simulink model "base_reference"  (R2019a)
settings: Solver=ode23tb  StartTime=0.0  StopTime=60  RelTol=1e-3
model workspace (MAT data in the model file):
  A_mu = 10
  AxlIxx = 62.3745166667
  AxlM = 160
  B_reff = 8.386
  BattCapInit = 26
  BattChargeMax = 32.5
  BattChrgMax = -80000
  BattDischrgMax = 80000
  BattTempBp = [243.1 253.1 263.1 273.1 283.1 298.1 313.1]
  BrkPrsMax = 5000000
  CapLUTBp = [0 0.01 0.02 0.03 0.04 0.05 0.06 0.07 0.08 0.09 0.1 0.11 ... (101 elements, 1x101)]
  CapSOCBp = [0 0.2 0.4 0.6 0.8 1]
  ChrgLmt_bpt = [1 1 1 1 1 1 1 1 0.7 0.35 0]
  Cps = 2
  Cz = 5565.2246438
  CzWhlAxl = 11490.971257
  DCT_Param : struct (value not decoded)
  DLCXref = [0 6 7 14 33.5 34 42 50 60]
  DLCYref = [0 0 -4.5 -4 -3.75 1.5 0.5 0 0]
  D_reff = 0.25826
  DischrgLmt_bpt = [0 0.35 0.7 1 1 1 1 1 1 1 1]
  Downshift_Speeds = [9.5625 12.9375 16.3125 19.6875 23.0625 26.4375 29.8125 33.1875 36.5625 39.9375 43.3125 46.6875 ... (28 elements, 4x7)]
  EV_current = 200
  EV_motion = [20 4 0.8]
  EV_sf = 2000
  Em = [2.8 3.228 3.284 3.361 3.408 3.427 3.472 3.477 3.493 3.504 3.516 3.528 ... (101 elements, 1x101)]
  EngRevLim = 7000
  F0z = [2886 2907]
  F0zWhlAxl = 2907
  Fs = 0
  Fv = 0.0025
  Hmax = 0.25
  Jcomp = 0.0227
  Ki = 251.3274
  Kisa = 346.6583
  Kp_d = 0.47149
  Kp_q = 0.52125
  Ksa = 85.4316
  Ksf = 1996.2651
  Kz = 52451.0065793
  KzWhlAxl = 138031.612078
  Ld = 0.0003752
  Ldq = [0.0003752 0.0004148]
  Lq = 0.0004148
  Mechanical = [0.0227 0.0025 0]
  MotMapEff = 0
  MotSpd = [0 1000 2000 2728.370453 3000 4000 5000 6000 7000 8000 9000 10000]
  MotTrq = [280 280 280 280 254.6479089 190.9859317 152.7887454 127.3239545 109.1348181 95.49296586 84.88263632 76.39437268]
  NCyl = 6
  Ndiff = 7.94
  Np = 2
  Ns = 96
  P = 4
  Pedal_Positions = [0.1 0.4 0.5 0.9]
  PolePairs = 4
  Pstd = 101325
  RInt = [0.008846 0.006389 0.004364 0.002031 0.001443 0.0005603 0.001028 0.009319 0.006554 0.004101 0.002563 0.001825 ... (42 elements, 7x6)]
  Rair = 287
  RegenBrkCutOff = [0 1]
  RegenBrkSpd_bpt = [5 9]
  Rm = 0.15
  Rs = 0.2
  SOC_bpt = [0 10 20 30 40 50 60 70 80 90 100]
  SUS : struct (value not decoded)
  T_eff_bp = [0 20 40 60 80 100 120 140 160 180 200 220 ... (15 elements, 1x15)]
  T_max = 120
  T_mtpa = [0 13.3131834767 26.6278836885 39.9456159322 53.2678926341 66.5962219318 79.9321062746 93.277041051 106.632513247 120.000000141]
  Tc = 0.02
  Trans : struct (value not decoded)
  Tstd = 293.15
  Upshift_Speeds = [12.9375 16.3125 19.6875 33 26.4375 29.8125 33.1875 52.5 39.9375 43.3125 46.6875 77.25 ... (28 elements, 4x7)]
  VEH : struct (value not decoded)
  V_o = 16.7
  V_xlow = 1
  Vd = 0.00346
  WH : struct (value not decoded)
  a = 1.4
  alpha_max = 1.5
  alpha_min = -1.5
  b = 1.8
  ba = 3.4029
  c_zo = 209651
  disk_abore = 0.05
  dt3D = 0.05
  efficiency_table = [85 85 85 85 85 85 85 85 85 85 85 85 ... (180 elements, 12x15)]
  epsilon = 0.1
  f_air = [0 0 0 0 0 0 0 0 0 0 0 0 ... (256 elements, 16x16)]
  f_co = [0 0 0 0 0 0 0 0 0 0 0 0 ... (256 elements, 16x16)]
  f_co2 = [0 0 0 0 0 0 0 0 0 0 0 0 ... (256 elements, 16x16)]
  f_eff = [352.135682859 352.135682859 320.724378192 303.655312657 295.930136708 291.240087194 291.240271258 291.240312459 291.240275452 291.240198499 291.240100781 291.240018769 ... (256 elements, 16x16)]
  f_fuel = [0 0 0 0 0 0 0 0 0 0 0 0 ... (256 elements, 16x16)]
  f_hc = [0 0 0 0 0 0 0 0 0 0 0 0 ... (256 elements, 16x16)]
  f_nox = [0 0 0 0 0 0 0 0 0 0 0 0 ... (256 elements, 16x16)]
  f_pm = [0 0 0 0 0 0 0 0 0 0 0 0 ... (256 elements, 16x16)]
  f_susp_axl_bp = [1 2]
  f_susp_dz_bp = [-0.325022776267 -0.315022776267 -0.305022776267 -0.205022776267 -0.105022776267 -0.00502277626717 0.0949772237328 0.194977223733 0.204977223733 0.214977223733]
  f_susp_dzdot_bp = [-3 -0.3 -0.2 -0.1 0 0.1 0.2 0.3 3]
  f_susp_fmz = [-144070.391448 -93629.24037 -75929.1118915 -20630.5828179 -15385.48216 -10140.3815021 -4895.28084414 349.819813785 -31916.3973792 18437.6709544 -83996.1993354 -33555.0482577 ... (43920 elements, 10x9x61x2x4)]
  f_susp_geom = [0 0 0 0 0 0 0 0 0 0 0 0 ... (3660 elements, 10x61x2x3)]
  f_susp_strgdelta_bp = [-0.523598775598 -0.506145483078 -0.488692190558 -0.471238898038 -0.453785605519 -0.436332312999 -0.418879020479 -0.401425727959 -0.383972435439 -0.366519142919 -0.349065850399 -0.331612557879 ... (61 elements, 1x61)]
  f_tbrake = [0 76.8593923996 105.140482948 131.533638111 157.926793274 176.658631717 176.65727296 176.656856686 176.656879077 176.657093756 176.657404516 176.65772406 ... (256 elements, 16x16)]
  f_tbrake_n_bpt = [0 649.519052838 912.419621844 1175.32019085 1438.22075986 1701.12132886 1964.02189787 2226.92246687 2489.82303588 2752.72360489 3015.62417389 3278.5247429 ... (16 elements, 1x16)]
  f_tbrake_t_bpt = [0 34.6410161514 61.0341713143 87.4273264773 113.82048164 140.213636803 166.606791966 192.999947129 219.393102292 245.786257455 272.179412618 298.572567781 ... (16 elements, 1x16)]
  f_texh = [766.752464599 766.752464599 786.17542386 801.679939032 884.591982581 910.574397722 910.571871054 910.570774534 910.570601632 910.570821151 910.571247242 910.571639815 ... (256 elements, 16x16)]
  f_twc_eff_co = [0.17 0.25 0.45 0.99 0.99 0.99 0.99]
  f_twc_eff_hc = [0.21 0.375 0.75 0.98 0.98 0.98 0.98]
  f_twc_eff_lam = [0.909090909 0.944055944 0.979020979 1 1.013986014 1.048951049 1.083916084]
  f_twc_eff_nox = [0.98 0.98 0.98 0.97 0.05 0.02 0]
  h = 0.134
  id_mtpa = [0 -0.114523352646 -0.457989076459 -1.03008464374 -1.83029075221 -2.85788367342 -4.11193850568 -5.59133329791 -7.29475400168 -9.22070020138]
  idq0 = [0 0]
  idq_limits = [-9.220699542 166.993501392 167.247872355]
  iq_mtpa = [0 18.5827440345 37.1633719111 55.7397734896 74.3098506185 92.871523015 111.422734008 129.961456105 148.485696337 166.993501356]
  lambda_pm = 0.1194
  mechanical = [0.0227 0.0025 0]
  mu_kinetic = 0.35
  numWheel = 4
  num_pads = 2
  omega_init = 0
  path : struct (value not decoded)
  pio = 220000
  power_max = 80000
  q_Fcx = 0
  q_Fz2 = 15.4
  q_Fzy = 0
  q_reo = 0.9974
  q_sx1 = -0.007764
  q_sx10 = 0.2824
  q_sx11 = 5.349
  q_sx12 = 0
  q_sx13 = 0
  q_sx14 = 0
  q_sx2 = 1.1915
  q_sx3 = 0.013948
  q_sx4 = 4.912
  q_sx5 = 1.02
  q_sx6 = 22.83
  q_sx7 = 0.7104
  q_sx8 = -0.023393
  q_sx9 = 0.6581
  q_sy1 = 0.00702
  q_sy2 = 0
  q_sy3 = 0.001515
  q_sy4 = 8.514e-05
  q_sy5 = 0
  q_sy6 = 0
  q_sy7 = 0.9008
  q_sy8 = -0.4089
  q_v1 = 0.0007742
  q_v2 = 0.04667
  r_Bx1 = 12.531
  r_Bx2 = 9.532
  r_Bx3 = 0
  r_By1 = 10.615
  r_By2 = 7.705
  r_By3 = 3.433e-06
  r_By4 = 0
  r_Cx1 = 1.019
  r_Cy1 = 1.0585
  r_Ex1 = -0.4487
  r_Ex2 = -0.4726
  r_Ey1 = 0.3132
  r_Ey2 = 7.63e-06
  r_Hx1 = 0.0002374
  r_Hy1 = 0.011646
  r_Hy2 = 7.63e-06
  r_Vy1 = 0.05654
  r_Vy2 = 7.63e-06
  r_Vy3 = 0
  r_Vy4 = 99.9
  r_Vy5 = 2
  r_Vy6 = 15.814
  r_o = 0.3135
  theta_init = 0
  torque_max = 280
  vehWidth = 2
  w = 1
  w_eff_bp = [0 1000 2000 2728.370453 3000 4000 5000 6000 7000 8000 9000 10000]
values from neighbouring files (symbols this model uses):
  VEH =     [PassVeh14DOF.mat]    (also in model2.mat; model_workspace_reference.mat)
undefined symbols (not defined in the file or in its folder): Disabled, Right
libraries: simulink x8, vehdynlibtire x8, vehdynlibsuspension x7, autolibutils x6, vehdynlibscenariocommon x5, sim3dlib x4, autolibmappedmotor x4, autolibshared x2, sharedtransform x2, vehdynlibviscommon x2, vehdynlibdriver x1, vehdynlibsteering x1
(part 2 of 8)

== system base_reference/Controllers ==
  Driver : Inport
  Vehicle_loop : Inport  Port=2
  Accel Pedal to Traction Wheel Torque Request : Subsystem
  Active Differential Control : Subsystem  VariantControlMode=Label  Variant=on  LabelModeActiveChoice=0
  Battery Management System : Subsystem
  Brake Pedal to Total Braking Pressure Request : Subsystem
  Bus Creator2 : BusCreator  Inputs=1
  Bus Creator3 : BusCreator  Inputs=3
  Bus Creator4 : BusCreator  Inputs=1
  Bus Selector : BusSelector  OutputSignals=ElecFdbk.BattSoc,Driveline.EngSpd,Body.r
  Bus Selector3 : BusSelector  OutputSignals=Steer,Accel,Brake
  Constant : Constant  Value=0
  Max : MinMax  Function=max  Inputs=2
  Motor Torque Arbitration and Power Management : Subsystem
  Regen Braking Control : Subsystem  VariantControlMode=Label  Variant=on  VariantControl=(default)  LabelModeActiveChoice=Variant
  Controller : Outport
  wires:
  Driver/1 -> Bus Selector3/1
  Max/1 -> Bus Creator3/1  "acc"
  Bus Creator2/1 -> Bus Creator3/2  "Brake"
  Bus Creator3/1 -> Controller/1  "Controller"
  Active Differential Control/1(DiffPrsCmd) -> Bus Creator4/1  "PrsCmd"
  Bus Selector3/1 -> Active Differential Control/2(Steer)  "<Steer>"
  Active Differential Control/2(TrqCmd) -> [DiffTrqCmd]
  Battery Management System/1(BattPwrDischrgLmt) -> Motor Torque Arbitration and Power Management/3(BattPwrDisChrgLmt)  "BattPwrDischrgLmt"
  Regen Braking Control/1(" MotTrqCmdRegen") -> Motor Torque Arbitration and Power Management/6(MotTrqCmdRegen)  "MotTrqCmdRegen"
  [MotSpd] -> Motor Torque Arbitration and Power Management/5(MotSpd)
  Bus Selector/2 -> Regen Braking Control/3("MotSpd "), [MotSpd], Regen Braking Control/2("VehSpd ")  "<EngSpd>"
  Accel Pedal to Traction Wheel Torque Request/1(TrqCmd) -> Motor Torque Arbitration and Power Management/1(MotTrqCmdTrac)
  Battery Management System/2(BattPwrChrgLmt) -> Motor Torque Arbitration and Power Management/4("BattPwrChrgLmt ")  "BattPwrChrgLmt"
  Bus Selector3/3 -> Brake Pedal to Total Braking Pressure Request/1(DecelPdl)  "<Brake>"
  Regen Braking Control/2(" BrkCmd") -> Bus Creator2/1  "BrkCmd"
  Constant/1 -> Brake Pedal to Total Braking Pressure Request/2(Park)
  [MotSpd] -> Accel Pedal to Traction Wheel Torque Request/2(MotSpd)
  Bus Selector/1 -> Battery Management System/1(SOC), Regen Braking Control/1("BattSoc ")  "<BattSoc>"
  Brake Pedal to Total Braking Pressure Request/1(BrkPrsReq) -> Regen Braking Control/4("BrkPrsReq ")
  [AccelPdl] -> Motor Torque Arbitration and Power Management/2(AccelPdl)
  Bus Selector3/2 -> [AccelPdl], Accel Pedal to Traction Wheel Torque Request/1(AccelPdl)  "<Accel>"
  Bus Creator4/1 -> Bus Creator3/3  "Diff"
  Vehicle_loop/1 -> Bus Selector/1
  Bus Selector/3 -> Active Differential Control/1(YawRate)  "<r>"
  [DiffTrqCmd] -> Max/1
  Motor Torque Arbitration and Power Management/1(MotTrqCmdFinal) -> Max/2  "MotTrqCmd4"

== system base_reference/Driver Commands ==
  VehRef : Inport
  VehFdbk : Inport  Port=2
  AccelGround : Ground
  BrakeGround : Ground
  Driver Commands : Subsystem  VariantControlMode=Label  Variant=on  VariantControl=Variant1  LabelModeActiveChoice=1  AllowZeroVariantControls=on
  GearGround : Ground
  SteerGround : Ground
  Driver : Outport
  wires:
  VehRef/1 -> Driver Commands/1(VehRef)
  VehFdbk/1 -> Driver Commands/2(VehFdbk)
  Driver Commands/1(" Driver") -> Driver/1
  SteerGround/1 -> Driver Commands/3(SteerCmd)
  AccelGround/1 -> Driver Commands/4(Accel)
  BrakeGround/1 -> Driver Commands/5(Brake)
  GearGround/1 -> Driver Commands/6(Gear)

== system base_reference/Environment ==
  Bus Creator1 : BusCreator  Inputs=4
  Constant3 : Constant  Value=0
  Constant4 : Constant  Value=0
  Constant5 : Constant  Value=0
  Constant6 : Constant  Value=300
  Constant7 : Constant  Value=101325
  Friction : Constant  Value=ones(4,1).*1
  Ground Feedback : Subsystem  VariantControlMode=Label  Variant=on  LabelModeActiveChoice=0
  Vector Concatenate : Concatenate  NumInputs=3
  Env : Outport
  wires:
  Constant5/1 -> Vector Concatenate/3  "Z"
  Vector Concatenate/1 -> Bus Creator1/3  "Wind"
  Constant3/1 -> Vector Concatenate/1  "X"
  Constant4/1 -> Vector Concatenate/2  "Y"
  Ground Feedback/1(Ground) -> Bus Creator1/4  "Gnd"
  Bus Creator1/1 -> Env/1
  Friction/1 -> Ground Feedback/1(Friction)
  Constant6/1 -> Bus Creator1/1  "Temp"
  Constant7/1 -> Bus Creator1/2  "Baro"

== system base_reference/Passenger Vehicle ==
  Env : Inport
  Operator : Inport  Port=2
  Cntrl : Inport  Port=3
  Bus Creator2 : BusCreator  Inputs=4
  Subsystem : Subsystem
  Subsystem1 : Subsystem
  Subsystem2 : Subsystem
  Subsystem4 : Subsystem
  Subsystem5 : Subsystem
  Subsystem6 : Subsystem
  VehFdbk : Outport
  wires:
  Bus Creator2/1 -> VehFdbk/1
  Env/1 -> Subsystem2/4(Env), Subsystem/1(Env)
  Subsystem1/1(Driveline) -> [Driveline], Bus Creator2/1  "Driveline"
  Subsystem5/1(WhlAng) -> Subsystem1/1(WhlAng)
  Operator/1 -> Subsystem2/2(SteerCmd)
  Cntrl/1 -> Subsystem2/1(Cntrl)
  Subsystem2/1(Steer) -> Subsystem5/1(SteerHWCmd)
  Subsystem2/2(brake) -> Subsystem5/2(BrkPrsCmd)
  Subsystem4/2(Wheels) -> Bus Creator2/4, [Wheels]  "Wheels"
  [Driveline] -> Subsystem/2(Driveline)
  [Wheels] -> Subsystem2/3(Wheels)
  Subsystem6/15(dzWheel) -> Subsystem4/15(dzWheel)
  Subsystem6/3(CgXYZdot) -> Subsystem4/3(CgXYZdot)
  Subsystem6/1(Cgxyzdot) -> Subsystem4/1(Cgxyzdot)
  Subsystem6/5(pqr) -> Subsystem4/5(pqr)
  Subsystem6/14(YWheel) -> Subsystem4/14(YWheel)
  Subsystem6/7(Beta) -> Subsystem4/7(Beta)
  Subsystem6/6(Cgaxyz) -> Subsystem4/6(Cgaxyz)
  Subsystem6/8(GeomXYZ) -> Subsystem4/8(GeomXYZ)
  Subsystem6/4(angles) -> Subsystem4/4(angles)
  Subsystem6/11(kappa) -> Subsystem4/11(kappa)
  Subsystem6/13(XWheel) -> Subsystem4/13(XWheel)
  Subsystem6/2(CgXYZ) -> Subsystem4/2(CgXYZ)
  Subsystem6/9(GeomXYZdot) -> Subsystem4/9(GeomXYZdot)
  Subsystem6/10(omega) -> Subsystem4/10(omega)
  Subsystem6/12(alpha) -> Subsystem4/12(alpha)
  Subsystem5/2(BrkPrs) -> Subsystem1/2(BrkPrs)
  Subsystem5/5(BattSoc) -> Subsystem1/5(BattSoc)
  Subsystem5/6(BattPwr) -> Subsystem1/6(BattPwr)
  Subsystem5/7(BattCrnt) -> Subsystem1/7(BattCrnt)
  Subsystem2/4(acc) -> Subsystem5/4("acc ")
  Subsystem5/3(AxlTrq) -> Subsystem1/3(AxlTrq)
  Subsystem5/4(Motor_speed) -> Subsystem1/4(EngSpd)
  Subsystem2/5(amb_temp) -> Subsystem5/5(AmbTmp)
  Subsystem2/3(omega) -> Subsystem5/3(speed_wheel)
  Subsystem1/2(ElecFdbk) -> Bus Creator2/2  "ElecFdbk"
  Subsystem4/1(Chassis) -> Bus Creator2/3  "Body"
  Subsystem/1(Wind) -> Subsystem6/1(WindXYZ)
  Subsystem/2(Gnd) -> Subsystem6/2(Ground)
  Subsystem/3(mu) -> Subsystem6/3(Friction)
  Subsystem/4(WhlAng) -> Subsystem6/4(WheelAngle)
  Subsystem/5(AxleTrq) -> Subsystem6/5(AxleTrq)
  Subsystem/6(BrkPrs) -> Subsystem6/6(BrkPrs)

== system base_reference/Reference Generator ==
  "VehFdbk " : Inport
  3D Engine : Subsystem  VariantControlMode=Label  Variant=on  LabelModeActiveChoice=0  mask(3D Engine){engine3D=Disabled, SceneDesc=Open surface, dt3D=dt3D, defaultPos=User-specified, X_o=X_o, Y_o=Y_o, Z_o=Z_o, phi_o=phi_o, theta_o=theta_o, psi_o=psi_o}
      mask prompts: engine3D "3D Engine"; SceneDesc "Scene:"; dt3D "Engine frame rate, dt3D [s]:"; X_o "Initial longitudinal position, X_o [m]:"; Y_o "Initial lateral position, Y_o [m]:"; Z_o "Initial vertical position, Z_o [m]:"; phi_o "Initial roll angle, phi_o [rad]:"; theta_o "Initial pitch angle, theta_o [rad]:"; psi_o "Initial yaw angle, psi_o [rad]:"
      mask help: This subsystem contains the interface blocks which permit the display of the vehicle in the 3D virtual environment. Enable it to view the simulation progress, disable it to inhibit the display.
      mask init:
      | switch get_param(gcb,'engine3D')
      |     case 'Disabled'
      |         set_param(gcb,'OverrideUsingVariant','0')
      |         try
      |             set_param([bdroot '/Environment/Ground Feedback'],'OverrideUsingVariant','0')
      |         catch
      |             disp('Warning: No ground feedback sensor not set')
      |         end
      |     case 'Enabled'
      |         set_param(gcb,'OverrideUsingVariant','1')
      |         try
      |             set_param([bdroot '/Environment/Ground Feedback'],'OverrideUsingVariant','1')
      |         catch
      |             disp('Warning: No ground feedback sensor not set')
      |         end
      |     otherwise
      |         set_param(gcb,'OverrideUsingVariant','0')
      | end
      settings: AttributesFormatString=|
      | %<SceneDesc>
      | %<engine3D>
      mask Help: eval('vdynblkshelp(''vdynblks3dengine'')');
      mask TypeOptions engine3D: Enabled | Disabled
      mask Callback engine3D:
      | switch get_param(gcb,'engine3D')
      |     case 'Disabled'
      |         set_param(gcb,'OverrideUsingVariant','0')
      |     case 'Enabled'
      |        set_param(gcb,'OverrideUsingVariant','1')
      |     otherwise
      |        set_param(gcb,'OverrideUsingVariant','0')
      | end
      mask TypeOptions SceneDesc:
      | 3D Engine/Simulation 3D Engine
      | 1/SceneDesc
      mask Callback SceneDesc: [~] = vdynblks3Dsceneconfig(gcb);
      mask TypeOptions defaultPos: Recommended for scene | User-specified
      mask DialogControl engineConfig Prompt: 3D Engine Settings
      mask DialogControl posSetup Prompt: Initial vehicle position
      mask DialogControl posSetupDesc Prompt: To use these initial vehicle positions, first Apply the initial values and then click Update the model workspaces with the initial values.
      mask DialogControl setModelPos Prompt: Update model workspaces with initial values
      mask DialogControl setModelPos Callback: [~] = vdynblksmdlWSconfig(gcb);
      mask Display: disp('3D Engine')
  Reference Generator : Subsystem  VariantControlMode=Label  Variant=on  VariantControl=Variant1  LabelModeActiveChoice=4
  " Vis" : Outport
  " Ref" : Outport  Port=2
  " Fdbk" : Outport  Port=3
  wires:
  "VehFdbk "/1 -> 3D Engine/1(VehFdbk), Reference Generator/1("VehFdbk ")
  Reference Generator/1(" Vis") -> " Vis"/1
  Reference Generator/2(" Ref") -> " Ref"/1
  Reference Generator/3(" Fdbk") -> " Fdbk"/1

== system base_reference/Visualization ==
  note: Vehicle Response
  note: Driver Commands
  Vis : Inport
  Cntrl : Inport  Port=2
  VehFdbk : Inport  Port=3
  Acceleration Cmd : LinearGaugeBlock  LabelPosition=Hide  ScaleMax=1  TickInterval=0.20000000000000001
  Brake Cmd : LinearGaugeBlock  LabelPosition=Hide  ScaleMax=1  TickInterval=0.20000000000000001
  Bus Selector : BusSelector  OutputSignals=Body.xdot,Body.ay
  Bus Selector2 : BusSelector  OutputSignals=Accel,Brake,Steer
  Engine Tach [rpm] : CircularGaugeBlock  LabelPosition=Hide  ScaleMax=8000  TickInterval=1000
  Handwheel Angle [deg] : SemiCircularGaugeBlock  LabelPosition=Hide  ScaleMin=-300  ScaleMax=300  TickInterval=60
  ISO 15037-1:2006 : Subsystem  StopFcn=|  VariantControlMode=Label  Variant=on  LabelModeActiveChoice=0  mask(ISO 15037-1:2006){Measurement=Disabled}
      | switch get_param(gcb,'Measurement')
      |     case 'Enabled'
      |        p=slproject.getCurrentProject;
      |        projectRoot=p.RootFolder;
      |        SySFolder=fullfile(projectRoot, 'System');
      |        Simulink.sdi.loadView([SySFolder filesep 'ISO15037_1_2006E.mldatx']);
      |        Simulink.sdi.view;
      | end
      mask prompts: Measurement "ISO Measurements"
      mask help: Enables display of ISO 15037-1:2006 standard measurement signals in the Simulation Data Inspector.
      mask init:
      | switch get_param(gcb,'Measurement')
      |     case 'Disabled'
      |         set_param(gcb,'OverrideUsingVariant','0')
      |     case 'Enabled'
      |        set_param(gcb,'OverrideUsingVariant','1')
      |     otherwise
      |        set_param(gcb,'OverrideUsingVariant','0')
      | end
      settings: AttributesFormatString=%<Measurement>
      mask Help: eval('vdynblkshelp(''iso15037'')');
      mask TypeOptions Measurement: Enabled | Disabled
      mask Callback Measurement:
      | switch get_param(gcb,'Measurement')
      |     case 'Disabled'
      |         set_param(gcb,'OverrideUsingVariant','0')
      |     case 'Enabled'
      |        set_param(gcb,'OverrideUsingVariant','1')
      |     otherwise
      |        set_param(gcb,'OverrideUsingVariant','0')
      | end
      mask Display: disp('ISO 15037-1:2006')
  Lateral Acceleration [g] : SemiCircularGaugeBlock  LabelPosition=Hide  ScaleMin=-1  ScaleMax=1  TickInterval=0.5
  Rate Transition1 : RateTransition  Deterministic=off  OutPortSampleTime=.1
  Rate Transition2 : RateTransition  Deterministic=off  OutPortSampleTime=.1
  Scope Type : Subsystem  VariantControlMode=Label  Variant=on  VariantControl=Variant1  LabelModeActiveChoice=2
  Signal Specification : SignalSpecification  Unit=deg
  Signal Specification1 : SignalSpecification  Unit=mph
  Speed [mph] : CircularGaugeBlock  LabelPosition=Hide  TickInterval=10
  Steer vs Ay : simulink/Sinks/XY Graph  Commented=on  xmin=-300  xmax=300  ymin=-1.5  ymax=1.5  st=.1
  "Steer, Velocity, Lat Accel" : Scope  NumInputPorts=3
  Terminator : Terminator
  Terminator1 : Terminator
  Terminator2 : Terminator
  Unit Conversion1 : UnitConversion
  Unit Conversion2 : UnitConversion
  Vehicle XY Plotter : Subsystem  VariantControlMode=Label  Variant=on  VariantControl=Variant1  LabelModeActiveChoice=1
  wires:
  Signal Specification/1 -> Rate Transition1/1, "Steer, Velocity, Lat Accel"/1  "SteerAngle"
  Bus Selector/2 -> Rate Transition2/1, "Steer, Velocity, Lat Accel"/3  "<ay>"
  Bus Selector/1 -> "Steer, Velocity, Lat Accel"/2, Unit Conversion1/1  "<xdot>"
  Unit Conversion2/1 -> Signal Specification/1
  Unit Conversion1/1 -> Signal Specification1/1
  Signal Specification1/1 -> Terminator/1  "xdot_mph"
  Bus Selector2/3 -> Unit Conversion2/1  "<Steer>"
  Rate Transition1/1 -> Steer vs Ay/1
  Rate Transition2/1 -> Steer vs Ay/2
  Bus Selector2/1 -> Terminator1/1  "<Accel>"
  Bus Selector2/2 -> Terminator2/1  "<Brake>"
  VehFdbk/1 -> ISO 15037-1:2006/1(VehFdbk), Scope Type/1("VehFdbk "), Vehicle XY Plotter/1("VehFdbk "), Bus Selector/1  "VehFdbk"
  Cntrl/1 -> ISO 15037-1:2006/2(Cntrl), Scope Type/2(Cntrl), Bus Selector2/1
  Vis/1 -> Scope Type/3("Vis ")
  Scope Type/1(" Ref") -> Vehicle XY Plotter/2("Ref ")

== system base_reference/Controllers/Accel Pedal to Traction Wheel Torque Request ==
  note: Convert Accelerator Pedal Position to Torque Command
      | using Motor Torque Speed Curve
  AccelPdl : Inport
  MotSpd : Inport  Port=2
  MaxMotTrqVsSpd : Lookup_n-D  NumberOfTableDimensions=1  BreakpointsForDimension1=MotSpd  Table=MotTrq  ExtrapMethod=Clip  UseLastTableValue=on  InternalRulePriority=Speed  OutDataTypeStr=Inherit: Inherit from 'Table data'  RndMeth=Simplest  InputSameDT=on
  Product1 : Product
  rads_to_rpm : Gain  Gain=30/pi
  TrqCmd : Outport
  wires:
  Product1/1 -> TrqCmd/1
  MaxMotTrqVsSpd/1 -> Product1/2
  AccelPdl/1 -> Product1/1
  MotSpd/1 -> rads_to_rpm/1
  rads_to_rpm/1 -> MaxMotTrqVsSpd/1

== system base_reference/Controllers/Active Differential Control ==
  note: 1) Add Subsystem or Model blocks as valid variant choices.
      | 2) You cannot connect blocks at this level. At simulation, connectivity is automatically
      | determined, based on the active variant and port name matching.
  YawRate : Inport
  Steer : Inport  Port=2
  No Control : Subsystem  VariantControl=0
  Rear Diff Controller : Subsystem  VariantControl=1
  DiffPrsCmd : Outport
  TrqCmd : Outport  Port=2

== system base_reference/Controllers/Battery Management System ==
  note: Behaviorial BMS System. Limits battery charge / discharge power based on SOC.
      |
      | Charge/Discharge Limits and curves can be adjusted if using a larger battery pack
      | or motor power is changed.
  SOC : Inport
  ChrgLmt : Lookup_n-D  NumberOfTableDimensions=1  BreakpointsForDimension1=SOC_bpt  Table=ChrgLmt_bpt  ExtrapMethod=Clip  UseLastTableValue=on  InternalRulePriority=Speed  RndMeth=Simplest  InputSameDT=on
  DischrgLmt : Lookup_n-D  NumberOfTableDimensions=1  BreakpointsForDimension1=SOC_bpt  Table=DischrgLmt_bpt  ExtrapMethod=Clip  UseLastTableValue=on  InternalRulePriority=Speed  RndMeth=Simplest  InputSameDT=on
  MaxChrg : Constant  Value=BattChrgMax
  MaxDischrg : Constant  Value=BattDischrgMax
  Product : Product
  Product1 : Product
  BattPwrDischrgLmt : Outport
  BattPwrChrgLmt : Outport  Port=2
  wires:
  SOC/1 -> DischrgLmt/1, ChrgLmt/1
  MaxChrg/1 -> Product1/2
  MaxDischrg/1 -> Product/2
  Product/1 -> BattPwrDischrgLmt/1
  Product1/1 -> BattPwrChrgLmt/1
  ChrgLmt/1 -> Product1/1
  DischrgLmt/1 -> Product/1

== system base_reference/Controllers/Brake Pedal to Total Braking Pressure Request ==
  note: Converts Brake Pedal Position to Brake Pressure Request
  DecelPdl : Inport
  Park : Inport  Port=2
  Constant : Constant  Value=BrkPrsMax
  Constant1 : Constant
  Product1 : Product
  Switch : Switch  Criteria=u2 > Threshold
  BrkPrsReq : Outport
  wires:
  Constant/1 -> Product1/2
  Switch/1 -> Product1/1
  DecelPdl/1 -> Switch/3
  Constant1/1 -> Switch/1
  Product1/1 -> BrkPrsReq/1
  Park/1 -> Switch/2

== system base_reference/Controllers/Motor Torque Arbitration and Power Management ==
  MotTrqCmdTrac : Inport
  AccelPdl : Inport  Port=2
  BattPwrDisChrgLmt : Inport  Port=3
  "BattPwrChrgLmt " : Inport  Port=4
  MotSpd : Inport  Port=5
  MotTrqCmdRegen : Inport  Port=6
  Accel Decel Switch : Switch  Criteria=u2 > Threshold
  Compare To Constant : simulink/Logic and Bit Operations/Compare To Constant  relop=>  const=0  OutDataTypeStr=boolean
  Power Management : Subsystem
  MotTrqCmdFinal : Outport
  wires:
  AccelPdl/1 -> Compare To Constant/1
  MotTrqCmdRegen/1 -> Accel Decel Switch/3
  MotTrqCmdTrac/1 -> Accel Decel Switch/1
  Power Management/1(MotTrqCmdFinal) -> MotTrqCmdFinal/1
  Accel Decel Switch/1 -> Power Management/4(MotTrqCmd)
  BattPwrDisChrgLmt/1 -> Power Management/1(BattPwrDischrgLmt)
  "BattPwrChrgLmt "/1 -> Power Management/2(BattPwrChrgLmt)
  MotSpd/1 -> Power Management/3(MotSpd)
  Compare To Constant/1 -> Accel Decel Switch/2

== system base_reference/Controllers/Regen Braking Control ==
  "BattSoc " : Inport
  "VehSpd " : Inport  Port=2
  "MotSpd " : Inport  Port=3
  "BrkPrsReq " : Inport  Port=4
  Parallel Regen Braking : Subsystem  InitFcn=%[~]=autosharedicon('autolibutils',gcb,0);  VariantControl=(default)
  Series Regen Braking : Subsystem  InitFcn=%[~]=autosharedicon('autolibutils',gcb,0);  VariantControl=Variant
  " MotTrqCmdRegen" : Outport
  " BrkCmd" : Outport  Port=2

== system base_reference/Driver Commands/Driver Commands ==
  VehRef : Inport
  VehFdbk : Inport  Port=2
  SteerCmd : Inport  Port=3
  Accel : Inport  Port=4
  Brake : Inport  Port=5
  Gear : Inport  Port=6
  Longitudinal Driver : Subsystem  VariantControl=0
  Open Loop Constant Radius : Subsystem  VariantControl=2
  Predictive Driver : Subsystem  VariantControl=1
  " Driver" : Outport

== system base_reference/Environment/Ground Feedback ==
  note: 1) Add Subsystem or Model blocks as valid variant choices.
      | 2) You cannot connect blocks at this level. At simulation, connectivity is automatically
      | determined, based on the active variant and port name matching.
  Friction : Inport
  3D Engine : Subsystem  VariantControl=1
  Constant : Subsystem  VariantControl=0
  Ground : Outport

== system base_reference/Passenger Vehicle/Subsystem ==
  Env : Inport
  Driveline : Inport  Port=2
  Bus Selector1 : BusSelector  OutputSignals=Gnd.z.G_FL_z,Gnd.z.G_FR_z,Gnd.z.G_RL_z,Gnd.z.G_RR_z
  Bus Selector2 : BusSelector  OutputSignals=Wind
  Bus Selector3 : BusSelector  OutputSignals=Gnd.mu.mu_FL,Gnd.mu.mu_FR,Gnd.mu.mu_RL,Gnd.mu.mu_RR
  Bus Selector4 : BusSelector  OutputSignals=WhlAng,AxlTrq,BrkPrs
  Vector Concatenate : Concatenate  NumInputs=4
  Vector Concatenate1 : Concatenate  NumInputs=4
  Wind : Outport
  Gnd : Outport  Port=2
  mu : Outport  Port=3
  WhlAng : Outport  Port=4
  AxleTrq : Outport  Port=5
  BrkPrs : Outport  Port=6
  wires:
  Env/1 -> Bus Selector3/1, Bus Selector1/1, Bus Selector2/1
  Bus Selector2/1 -> Wind/1  "<Wind>"
  Bus Selector3/1 -> Vector Concatenate/1  "<mu_FL>"
  Bus Selector3/2 -> Vector Concatenate/2  "<mu_FR>"
  Bus Selector3/3 -> Vector Concatenate/3  "<mu_RL>"
  Bus Selector3/4 -> Vector Concatenate/4  "<mu_RR>"
  Vector Concatenate/1 -> mu/1
  Bus Selector1/1 -> Vector Concatenate1/1  "<G_FL_z>"
  Bus Selector1/2 -> Vector Concatenate1/2  "<G_FR_z>"
  Bus Selector1/3 -> Vector Concatenate1/3  "<G_RL_z>"
  Bus Selector1/4 -> Vector Concatenate1/4  "<G_RR_z>"
  Vector Concatenate1/1 -> Gnd/1
  Driveline/1 -> Bus Selector4/1
  Bus Selector4/2 -> AxleTrq/1  "<AxlTrq>"
  Bus Selector4/1 -> WhlAng/1  "<WhlAng>"
  Bus Selector4/3 -> BrkPrs/1  "<BrkPrs>"

== system base_reference/Passenger Vehicle/Subsystem1 ==
  WhlAng : Inport
  BrkPrs : Inport  Port=2
  AxlTrq : Inport  Port=3
  EngSpd : Inport  Port=4
  BattSoc : Inport  Port=5
  BattPwr : Inport  Port=6
  BattCrnt : Inport  Port=7
  Bus Creator1 : BusCreator  Inputs=4
  Bus Creator3 : BusCreator  Inputs=4
  Driveline : Outport
  ElecFdbk : Outport  Port=2
  wires:
  Bus Creator1/1 -> Driveline/1  "Driveline"
  AxlTrq/1 -> Bus Creator1/2, Bus Creator3/4  "AxlTrq"
  WhlAng/1 -> Bus Creator1/1  "WhlAng"
  EngSpd/1 -> Bus Creator1/4  "EngSpd"
  BrkPrs/1 -> Bus Creator1/3  "BrkPrs"
  BattCrnt/1 -> Bus Creator3/3
  BattPwr/1 -> Bus Creator3/2
  BattSoc/1 -> Bus Creator3/1
  Bus Creator3/1 -> ElecFdbk/1  "ElecFdbk"

== system base_reference/Passenger Vehicle/Subsystem2 ==
  Cntrl : Inport
  SteerCmd : Inport  Port=2
  Wheels : Inport  Port=3
  Env : Inport  Port=4
  Bus Selector1 : BusSelector  OutputSignals=Steer
  Bus Selector2 : BusSelector  OutputSignals=omega
  Bus Selector3 : BusSelector  OutputSignals=Brake,acc
  Bus Selector4 : BusSelector  OutputSignals=Temp
  Steer : Outport
  brake : Outport  Port=2
  omega : Outport  Port=3
  acc : Outport  Port=4
  amb_temp : Outport  Port=5
  wires:
  Cntrl/1 -> Bus Selector3/1
  SteerCmd/1 -> Bus Selector1/1
  Wheels/1 -> Bus Selector2/1
  Bus Selector2/1 -> omega/1  "<omega>"
  Bus Selector3/1 -> brake/1  "<Brake>"
  Bus Selector1/1 -> Steer/1  "<Steer>"
  Bus Selector3/2 -> acc/1  "<acc>"
  Bus Selector4/1 -> amb_temp/1  "<Temp>"
  Env/1 -> Bus Selector4/1

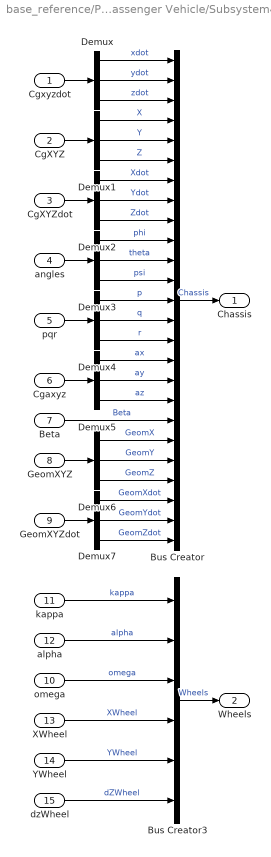
== system base_reference/Passenger Vehicle/Subsystem4 ==
  Cgxyzdot : Inport
  CgXYZ : Inport  Port=2
  CgXYZdot : Inport  Port=3
  angles : Inport  Port=4
  pqr : Inport  Port=5
  Cgaxyz : Inport  Port=6
  Beta : Inport  Port=7
  GeomXYZ : Inport  Port=8
  GeomXYZdot : Inport  Port=9
  omega : Inport  Port=10
  kappa : Inport  Port=11
  alpha : Inport  Port=12
  XWheel : Inport  Port=13
  YWheel : Inport  Port=14
  dzWheel : Inport  Port=15
  Bus Creator : BusCreator  Inputs=25
  Bus Creator3 : BusCreator  Inputs=6
  Demux{,1..7} (8 alike) : Demux  Outputs=3
  Chassis : Outport
  Wheels : Outport  Port=2
  wires:
  Bus Creator/1 -> Chassis/1  "Chassis"
  omega/1 -> Bus Creator3/3  "omega"
  dzWheel/1 -> Bus Creator3/6  "dZWheel"
  kappa/1 -> Bus Creator3/1  "kappa"
  Bus Creator3/1 -> Wheels/1  "Wheels"
  YWheel/1 -> Bus Creator3/5  "YWheel"
  XWheel/1 -> Bus Creator3/4  "XWheel"
  alpha/1 -> Bus Creator3/2  "alpha"
  Cgxyzdot/1 -> Demux/1
  CgXYZ/1 -> Demux1/1
  CgXYZdot/1 -> Demux2/1
  angles/1 -> Demux3/1
  pqr/1 -> Demux4/1
  Cgaxyz/1 -> Demux5/1
  GeomXYZdot/1 -> Demux7/1
  GeomXYZ/1 -> Demux6/1
  Demux/1 -> Bus Creator/1  "xdot"
  Demux/2 -> Bus Creator/2  "ydot"
  Demux/3 -> Bus Creator/3  "zdot"
  Demux1/1 -> Bus Creator/4  "X"
  Demux1/2 -> Bus Creator/5  "Y"
  Demux1/3 -> Bus Creator/6  "Z"
  Demux2/1 -> Bus Creator/7  "Xdot"
  Demux2/2 -> Bus Creator/8  "Ydot"
  Demux2/3 -> Bus Creator/9  "Zdot"
  Demux3/1 -> Bus Creator/10  "phi"
  Demux3/2 -> Bus Creator/11  "theta"
  Demux3/3 -> Bus Creator/12  "psi"
  Demux4/1 -> Bus Creator/13  "p"
  Demux4/2 -> Bus Creator/14  "q"
  Demux4/3 -> Bus Creator/15  "r"
  Demux5/1 -> Bus Creator/16  "ax"
  Demux5/2 -> Bus Creator/17  "ay"
  Demux5/3 -> Bus Creator/18  "az"
  Beta/1 -> Bus Creator/19  "Beta"
  Demux6/1 -> Bus Creator/20  "GeomX"
  Demux6/2 -> Bus Creator/21  "GeomY"
  Demux6/3 -> Bus Creator/22  "GeomZ"
  Demux7/1 -> Bus Creator/23  "GeomXdot"
  Demux7/2 -> Bus Creator/24  "GeomYdot"
  Demux7/3 -> Bus Creator/25  "GeomZdot"

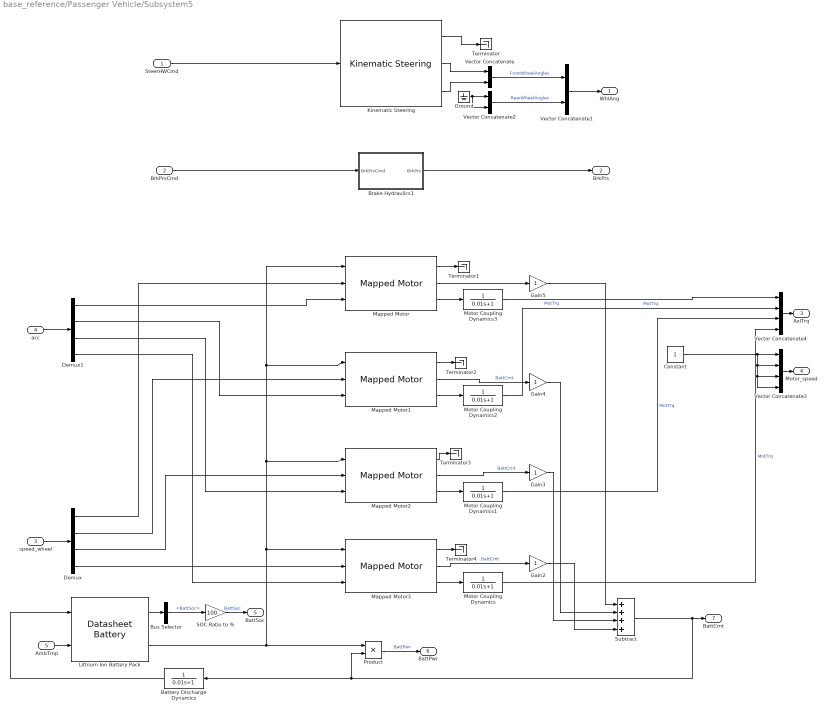
== system base_reference/Passenger Vehicle/Subsystem5 ==
  SteerHWCmd : Inport
  BrkPrsCmd : Inport  Port=2  PortDimensions=4
  speed_wheel : Inport  Port=3
  "acc " : Inport  Port=4
  AmbTmp : Inport  Port=5
  Battery Discharge Dynamics : TransferFcn  Denominator=[0.01 1]
  Brake Hydraulics1 : Subsystem
  Bus Selector : BusSelector  OutputSignals=BattSoc
  Constant : Constant
  Demux : Demux
  Demux1 : Demux
  Gain{2..5} (4 alike) : Gain
  Ground : Ground
  Kinematic Steering : vehdynlibsteering/Kinematic Steering  StrgType=Ackerman  StrgRatioType=Constant  Loc=Front  NrmlFctr=1  TrckWdth=1.922  WhlBase=(1.515+1.504)  Db=0  StrgRng=3*pi  StrgAngBpts="[-6.2832   -5.0265   -3.7699   -2.5133   -1.2566         0    1.2566    2.5133    3.7699    5.0265    6.2832]"  StrgRatioTbl=|  StrgRatio=18  StrgArmLngth=0.1  RckCsLngth=0.5  TieRodLngth=0.248128028933392  D=0.2  PnnRadius=0.0057  PnnRadiusTbl="[0.0055    0.0055    0.0056    0.0057    0.0057    0.0057    0.0057    0.0057    0.0056    0.0055    0.0055]"  RodLngth=0.1  ParaArmLngth=0.9  aMode=2
      | [13.5000   13.3750   13.2500   13.1250   13.0000   13.0000   13.0000   13.1250   13.2500   13.3750   13.5000
      | ]
      settings: SourceProductName=Vehicle Dynamics Blockset
  Lithium Ion Battery Pack : autolibdatasheetbattery/Datasheet Battery  CapacityCtrl=Parameter  OutputVlt=Unfiltered  BattChargeMax=BattChargeMax  Em=Em  CapLUTBp=CapLUTBp  RInt=RInt  BattTempBp=BattTempBp  CapSOCBp=CapSOCBp  Ns=Ns  Np=Np  BattCapInit=BattCapInit  Tc=1/1000  Vinit=3.75*72  RefBlkName='autolibdatasheetbattery/Datasheet Battery'
      settings: SourceProductName=Powertrain Blockset  SourceProductBaseCode=PW
  Mapped Motor{,1..3} (4 alike) : autolibmappedmotor/Mapped Motor  port_config=Speed  param_by=Maximum torque and power  w_t=[ 0 375 750 800 ]  T_t=[0.09 0.08 0.07 0]  torque_max=torque_max  power_max=power_max  Tc=Tc  param_loss=Tabulated efficiency data  eff=100  w_eff=375  T_eff=0.08  Piron=0  Pbase=0  w_eff_bp=w_eff_bp.*pi/30  T_eff_bp=T_eff_bp  Temp_eff_bp=[233.15 293.15 373.15]  losses_table=[1 2;3 4]  losses_table_3d=cat(3,[1.49 1.67 2.21 3.10; 0.42 0.69 1.14 2.03; 0.06 0.24 0.78 1.68; 0.42 0.69 1.14 2.03; 1.49 1.67 2.21 3.10],[1.49 1.67 2.21 3.10; 0.42 0.69 1.14 2.03; 0.06 0.24 0.78 1.68; 0.42 0.69 1.14 2.03; 1.49 1.67 2.21 3.10],[1.49 1.67 2.21 3.10; 0.42 0.69 1.14 2.03; 0.06 0.24 0.78 1.68; 0.42 0.69 1.14 2.03; 1.49 1.67 2.21 3.10])  efficiency_table=efficiency_table  efficiency_table_3d=cat(3,[95 95 95 95; 95 95 95 95; 95 95 95 95; 95 95 95 95; 95 95 95 95],[95 95 95 95; 95 95 95 95; 95 95 95 95; 95 95 95 95; 95 95 95 95],[95 95 95 95; 95 95 95 95; 95 95 95 95; 95 95 95 95; 95 95 95 95])  J=5e-6  b=1e-5  omega_o=0  T_t_extended=[0 0.07 0.08 0.09 0.08 0.07 0]  w_t_extended=[-800 -750 -375 0 375 750 800]  KLossIron=0  KLossCopper=0  x_w_eff_vec=[-1047.1975511966 -942.477796076938 -837.758040957278 -733.038285837618 -628.318530717959 -523.598775598299 -418.879020478639 -314.159265358979 -285.714285713875 -209.43951023932 -104.71975511966 0 104.71975511966 209.43951023932 285.714285713875 314.159265358979 418.879020478639 523.598775598299 628.318530717959 733.038285837618 837.758040957278 942.477796076938 1047.1975511966]  x_T_eff_vec=[-280 -260 -240 -220 -200 -180 -160 -140 -120 -100 -80 -60 -40 -20 0 20 40 60 80 100 120 140 160 180 200 220 240 260 280]  x_tmp_eff_vec=[-0.09 -0.06 -0.03 0 0.03 0.06 0.09]  x_losses_mat=[22069.9698961863 20493.5434750302 18917.117053874 17340.6906327178 15764.2642115617 14187.8377904055 12611.4113692493 11034.9849480932 9458.558526937 7882.13210578084 6305.70568462467 5463.63939754746 4654.21133865155 3695.99135716446 0 3141.59265358979 4188.79020478639 5026.54824574367 5864.30628670094 7330.38285837618 8796.45943005141 10262.5360017267 11728.6125734019 13194.6891450771 14660.7657167524 16126.8422884276 17592.9188601028 19058.9954317781 20525.0720034533;16844.2840149921 15641.1208710641 14437.9577271361 13234.7945832081 12031.6314392801 10828.4682953521 9625.30515142405 8422.14200749604 7218.97886356803 6015.81571964003 4812.65257571202 3609.48943178402 2837.5675580811 3326.39222144802 0 2827.43338823081 2638.93782901542 3392.92006587697 4523.8934211693 5654.86677646162 6785.84013175395 7916.81348704627 9047.7868423386 10178.7601976309 11309.7335529232 12440.7069082156 13571.6802635079 14702.6536188002 15833.6269740925;12345.907972002 11464.0574025733 10582.2068331446 9700.35626371584 8818.50569428713 7936.65512485842 7054.8045554297 6172.95398600099 5291.10341657228 4409.25284714356 3527.40227771485 3208.43505047468 2522.28227384987 2956.79308573157 0 2513.27412287184 2345.72251468038 3015.9289474462 3351.03216382911 4188.79020478639 5026.54824574366 5864.30628670094 6702.06432765822 7539.82236861549 8377.58040957277 9215.33845053005 10053.0964914873 10890.8545324446 11728.6125734019;10802.6694755017 10031.0502272516 9259.43097900148 8487.81173075136 7716.19248250124 6944.57323425111 6172.95398600099 5401.33473775087 4629.71548950074 3858.09624125062 3086.47699300049 2807.38066916535 2206.99698961863 2587.19395001512 0 2199.11485751286 2052.50720034533 2638.93782901542 2932.15314335047 3665.19142918809 4398.2297150257 5131.26800086332 5864.30628670094 6597.34457253856 7330.38285837617 8063.42114421379 8796.45943005141 9529.49771588903 10262.5360017266;9259.43097900149 8598.04305192995 7936.65512485842 7275.26719778688 6613.87927071535 5952.49134364381 5291.10341657228 4629.71548950074 3968.32756242921 3306.93963535767 3208.43505047468 2406.32628785601 1891.7117053874 2217.59481429868 0 1884.95559215388 1759.29188601028 2261.94671058465 3015.9289474462 3141.59265358979 3769.91118430775 4398.22971502571 5026.54824574366 5654.86677646162 6283.18530717958 6911.50383789754 7539.82236861549 8168.14089933345 8796.45943005141;7716.19248250124 7165.03587660829 6613.87927071535 6062.7226648224 5511.56605892946 4960.40945303651 4409.25284714356 3858.09624125062 3306.93963535767 2755.78302946473 2673.69587539557 2005.27190654668 1576.42642115617 1847.99567858223 0 1570.7963267949 1466.07657167524 1884.95559215387 2513.27412287183 2617.99387799149 3141.59265358979 3665.19142918809 4188.79020478639 4712.38898038468 5235.98775598298 5759.58653158128 6283.18530717958 6806.78408277788 7330.38285837618;7486.34845110759 6951.60927602848 6416.87010094936 5882.13092587025 5347.39175079114 4812.65257571202 4277.91340063291 3743.17422555379 3208.43505047468 2673.69587539557 2138.95670031645 1604.21752523734 1261.14113692493 1478.39654286579 0 1256.63706143592 1172.86125734019 1507.9644737231 2010.61929829747 2513.27412287183 3015.9289474462 3518.58377202056 4021.23859659493 4523.8934211693 5026.54824574366 5529.20307031803 6031.8578948924 6534.51271946676 7037.16754404113;9773.84381116825 9075.71211037052 8377.58040957279 7679.44870877505 5463.63939754746 4917.27545779272 4370.91151803797 3310.49548442795 2837.5675580811 2364.63963173425 1891.7117053874 1639.09181926424 1092.72787950949 1108.79740714934 0 942.477796076938 1005.30964914873 1507.9644737231 1759.29188601028 2199.11485751285 2638.93782901542 3078.760800518 4021.23859659493 4523.8934211693 5026.54824574367 6911.50383789754 7539.8223686155 8168.14089933346 8796.45943005142;8888.88888887612 8253.9682539564 7619.04761903668 6984.12698411695 4968.94409937174 4472.04968943457 3975.15527949739 3478.26086956022 2981.36645962304 2484.47204968587 1987.5776397487 ...(+6498 chars)]  x_losses_mat_3d=[37.8947368421052 25.2631578947368 12.6315789473684 0 12 24 36;18.9473684210526 12.6315789473684 6.3157894736842 0 5.99999999999999 12 18;0 0 0 0 0 0 0;18 12 5.99999999999999 0 6.3157894736842 12.6315789473684 18.9473684210526;36 24 12 0 12.6315789473684 25.2631578947368 37.8947368421052]  CalLossMapData={}  CalLossWithTempMapData={}  aMode=aMode  RefBlkName='autolibmappedmotor/Mapped Motor'
      settings: SourceProductName=Powertrain Blockset  SourceProductBaseCode=PW
  Motor Coupling Dynamics{,1..3} (4 alike) : TransferFcn  Denominator=[0.01 1]
  Product : Product
  SOC Ratio to % : Gain  Gain=100
  Subtract : Sum  Inputs=++++
  Terminator{,1..4} (5 alike) : Terminator
  Vector Concatenate : Concatenate
  Vector Concatenate1 : Concatenate
  Vector Concatenate2 : Concatenate
  Vector Concatenate3 : Concatenate  NumInputs=4
  Vector Concatenate4 : Concatenate  NumInputs=4
  WhlAng : Outport  Unit=rad
  BrkPrs : Outport  Port=2  PortDimensions=4
  AxlTrq : Outport  Port=3
  Motor_speed : Outport  Port=4
  BattSoc : Outport  Port=5
  BattPwr : Outport  Port=6
  BattCrnt : Outport  Port=7
  wires:
  SteerHWCmd/1 -> Kinematic Steering/1
  Kinematic Steering/1 -> Terminator/1
  Vector Concatenate2/1 -> Vector Concatenate1/2  "RearWheelAngles"
  Vector Concatenate1/1 -> WhlAng/1
  BrkPrsCmd/1 -> Brake Hydraulics1/1(BrkPrsCmd)
  Brake Hydraulics1/1(BrkPrs) -> BrkPrs/1
  Kinematic Steering/2 -> Vector Concatenate/1
  Kinematic Steering/3 -> Vector Concatenate/2
  Vector Concatenate/1 -> Vector Concatenate1/1  "FrontWheelAngles"
  Mapped Motor3/3 -> Motor Coupling Dynamics/1
  Battery Discharge Dynamics/1 -> Lithium Ion Battery Pack/1
  Product/1 -> BattPwr/1  "BattPwr"
  Motor Coupling Dynamics/1 -> Vector Concatenate4/4  "MotTrq"
  AmbTmp/1 -> Lithium Ion Battery Pack/2
  SOC Ratio to %/1 -> BattSoc/1  "BattSoc"
  Lithium Ion Battery Pack/2 -> Product/1, Mapped Motor3/1, Mapped Motor2/1, Mapped Motor1/1, Mapped Motor/1
  Demux1/4 -> Mapped Motor3/3
  Demux1/3 -> Mapped Motor2/3
  Mapped Motor2/3 -> Motor Coupling Dynamics1/1
  Motor Coupling Dynamics1/1 -> Vector Concatenate4/3  "MotTrq"
  Demux1/2 -> Mapped Motor1/3
  Motor Coupling Dynamics2/1 -> Vector Concatenate4/2  "MotTrq"
  Demux1/1 -> Mapped Motor/3
  Motor Coupling Dynamics3/1 -> Vector Concatenate4/1  "MotTrq"
  Vector Concatenate4/1 -> AxlTrq/1
  Subtract/1 -> Product/2, Battery Discharge Dynamics/1, BattCrnt/1
  Mapped Motor2/2 -> Gain3/1  "BattCrnt"
  Mapped Motor1/2 -> Gain4/1  "BattCrnt"
  Mapped Motor3/2 -> Gain2/1  "BattCrnt"
  Gain2/1 -> Subtract/4
  Gain3/1 -> Subtract/3
  Gain4/1 -> Subtract/2
  Gain5/1 -> Subtract/1
  "acc "/1 -> Demux1/1
  Mapped Motor/1 -> Terminator1/1
  Mapped Motor/3 -> Motor Coupling Dynamics3/1
  Mapped Motor/2 -> Gain5/1
  Mapped Motor1/3 -> Motor Coupling Dynamics2/1
  Mapped Motor1/1 -> Terminator2/1
  Mapped Motor2/1 -> Terminator3/1
  Mapped Motor3/1 -> Terminator4/1
  Vector Concatenate3/1 -> Motor_speed/1
  speed_wheel/1 -> Demux/1
  Demux/1 -> Mapped Motor/2
  Demux/2 -> Mapped Motor1/2
  Demux/3 -> Mapped Motor2/2
  Demux/4 -> Mapped Motor3/2
  Lithium Ion Battery Pack/1 -> Bus Selector/1
  Bus Selector/1 -> SOC Ratio to %/1  "<BattSoc>"
  Constant/1 -> Vector Concatenate3/1, Vector Concatenate3/2, Vector Concatenate3/3, Vector Concatenate3/4
  Ground/1 -> Vector Concatenate2/2, Vector Concatenate2/1
